simulink model "mcb_pmsm_param_est_host_f28379d"  (R2024b)
settings: Solver=FixedStepDiscrete  StartTime=0.0  StopTime=inf  RelTol=1e-3  EnableMultiTasking=on
StopFcn:
  | motorParam.p = motor.p;
  | motorParam.nomCurrent = motor.I_rated;
  | motorParam.PositionOffset = motor.PositionOffset;
  | motorParam.QEPSlits = motor.QEPSlits;
  | mcb_param_est_StopFunc(bdroot);
values from neighbouring files (symbols this model uses):
  Ts = T_pwm    (= 5e-05)    [mcb_pmsm_param_est_f28379d_data.m]
undefined symbols (not defined in the file or in its folder): motor
libraries: simulink x4, instrumentseriallib x3, mcbpmsmparamestlib x1
settings Model: Creator=The MathWorks, Inc.  LastModifiedBy=The MathWorks, Inc.
settings SolverCC: AlgebraicLoopSolver=TrustRegion
settings DataIOCC: LimitDataPoints=on  SaveFormat=Array  ReturnWorkspaceOutputs=off
settings OptimizationCC: ReuseModelBlockBuffer=off  LifeSpan=1  EfficientTunableParamExpr=on
settings DebuggingCC: UnderspecifiedInitializationDetection=Classic  MergeDetectMultiDrivingBlocksExec=none  SolverPrmCheckMsg=warning  ParameterPrecisionLossMsg=none  UnconnectedInputMsg=warning  UnconnectedOutputMsg=warning  UnconnectedLineMsg=warning  AllowSymbolicDim=off  PregeneratedLibrarySubsystemCodeDiagnostic=none  SubsystemReferenceDiagnosticForUnitTest=warning  SFUnexpectedBacktrackingDiag=warning  SFNoUnconditionalDefaultTransitionDiag=warning  SFExecutionAtInitializationDiag=none  ArithmeticOperatorsInVariantConditions=warning
settings HardwareCC: ProdBitPerPointer=32  ProdLargestAtomicFloat=None  ProdIntDivRoundTo=Undefined  ProdEndianess=Unspecified  ProdWordSize=32  ProdHWDeviceType=32-bit Generic
settings ModelReferenceCC: EnableRefExpFcnMdlSchedulingChecks=on  PropagateSignalLabelsOutOfModel=off
settings SFSimCC: SimUseLocalCustomCode=off  MATLABDynamicMemAlloc=off
settings RTWCC: Description=Real-Time Workshop Embedded Coder  SystemTargetFile=ert.tlc  TemplateMakefile=ert_default_tmf  GenerateReport=on  RTWUseLocalCustomCode=off  IncludeHyperlinkInReport=on  LaunchReport=on  GenerateTraceInfo=on  GenerateTraceReport=on  GenerateTraceReportSl=on  GenerateTraceReportSf=on  GenerateTraceReportEml=on  GPUComputeCapability=3.5  DLArmComputeVersion=19.05
settings CodeAppCC: IgnoreCustomStorageClasses=off  StateflowObjectComments=on  InternalIdentifier=Classic
settings ERTTargetCC: MultiwordLength=2048  GenerateSampleERTMain=on  InlinedParameterPlacement=Hierarchical  ERTCustomFileTemplate=example_file_process.tlc  ConvertIfToSwitch=off  SuppressUnreachableDefaultCases=off  DynamicArrayContainerType=coder::array
settings ConfigComp: CovMetricSettings=dw  CovSaveCumulativeToWorkspaceVar=on  CovSaveSingleToWorkspaceVar=on  CovExternalEMLEnable=off  CovSFcnEnable=off

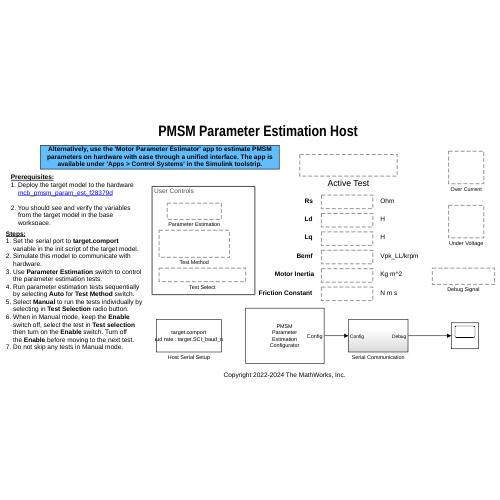
[thumbnail: Simulink's stored preview of the top-level diagram]
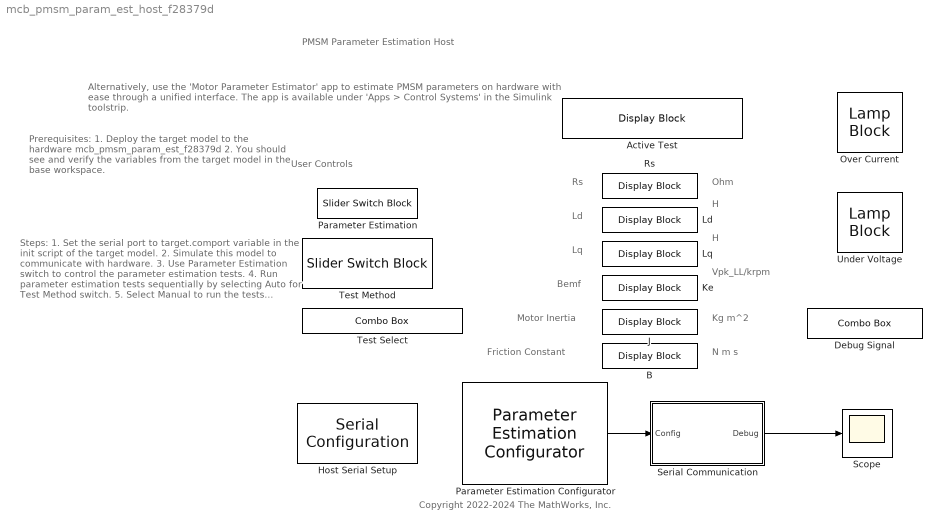
== system mcb_pmsm_param_est_host_f28379d ==
  note: Friction Constant
  note: User Controls
  note: PMSM Parameter Estimation Host
  note: Steps:
      | 1. Set the serial port to target.comport
      | variable in the init script of the target model.
      | 2. Simulate this model to communicate with
      | hardware.
      | 3. Use Parameter Estimation switch to control
      | the parameter estimation tests.
      | 4. Run parameter estimation tests sequentially
      | by selecting Auto for Test Method switch.
      | 5. Select Manual to run the tests individually by
      | selecting in Test Selection radio button.
      | 6. When in Manual mode, keep the Enable
      | switch off, select the test in Test selection
      | then turn on the Enable switch. Turn off
      | the Enable before moving to the next test.
      | 7. Do not skip any tests in Manual mode.
  note: H
  note: N m s
  note: Bemf
  note: Vpk_LL/krpm
  note: H
  note: Ohm
  note: Lq
  note: Rs
  note: Motor Inertia
  note: Copyright 2022-2024 The MathWorks, Inc.
  note: Ld
  note: Prerequisites:
      | 1. Deploy the target model to the hardware
      | mcb_pmsm_param_est_f28379d
      |
      | 2. You should see and verify the variables
      | from the target model in the base
      | workspace.
  note: Kg m^2
  note: Alternatively, use the 'Motor Parameter Estimator' app to estimate PMSM parameters on hardware with ease through a unified interface. The app is available under 'Apps > Control Systems' in the Simulink toolstrip.
  Active Test : DisplayBlock  LabelPosition=Hide  Transparency=1
  B : DisplayBlock  LabelPosition=Hide  Transparency=1
  Debug Signal : ComboBox  LabelPosition=Hide  SelectedLabel=Ia
      settings: Values={{'Ia', 'Ib', 'Vdc', 'Speed', 'Theta', 'Id', 'Iq', 'Vd', 'Vq', 'InjFreq', 'PhaseDiff', 'CoastDown Time'}, [1 2 3 4 5 6 7 8 9 10 11 12]}
  Host Serial Setup : instrumentseriallib/Serial Configuration  Priority=-99  PortSel=target.comport  Port=target.comport  ComPort=target.comport  BaudRate=target.SCI_baud_rate  DataBits=8  Parity=none  StopBits=1  ByteOrder=little-endian  FlowControl=none  Timeout=2  SimulateUsing=Interpreted execution  BlockInModel=on  aMode=5
      settings: LibrarySourceBlock=mcblib/Protection and Diagnostics/Host Serial Setup
  J : DisplayBlock  LabelPosition=Hide  Transparency=1
  Ke : DisplayBlock  LabelPosition=Hide  Transparency=1
  Ld : DisplayBlock  LabelPosition=Hide  Transparency=1
  Lq : DisplayBlock  LabelPosition=Hide  Transparency=1
  Over Current : LampBlock  LabelPosition=Hide
  Parameter Estimation : SliderSwitchBlock  LabelPosition=Hide
      settings: Values={{'Stop', 'Start'}, [0 1]}
  Parameter Estimation Configurator : mcbpmsmparamestlib/Parameter Estimation Configurator  P=motor.p  NRated=motor.N_rated  IRated=motor.I_rated  ImaxInverter=inverter.ISenseMax  RBoard=inverter.R_board  ISenseGain=0.0105  VSenseGain=0.0098  FreqMax=1000  FreqMin=400  FreqStepSweep=100  FreqStepEst=10  FreqNum=10  CurrMeasDelay=2 * 50e-6  KeTime=5  KeSpeed=0.9 * motor.N_rated  IqRefFOC=0.2  KpKiInputEnable=off  Kp=1  Ki=10  JSpeedLow=0.2 * motor.N_rated  DataType=single  Ts=Ts
      settings: LibrarySourceBlock=mcblib/Parameter Estimation/PMSM Parameter Estimation/Parameter Estimation Configurator
  Rs : DisplayBlock  LabelPosition=Hide  Transparency=1
  Scope : Scope
  Serial Communication : Subsystem
  Test Method : SliderSwitchBlock  LabelPosition=Hide
      settings: Values={{'Manual', 'Auto'}, [0 1]}
  Test Select : ComboBox  LabelPosition=Hide  SelectedLabel=No Test
      settings: Values={{'No Test', 'Rs', 'Ld', 'Lq', 'Ke, J, B'}, [0 1 2 3 4]}
  Under Voltage : LampBlock  LabelPosition=Hide
  wires:
  Serial Communication/1(Debug) -> Scope/1
  Parameter Estimation Configurator/1 -> Serial Communication/1(Config)

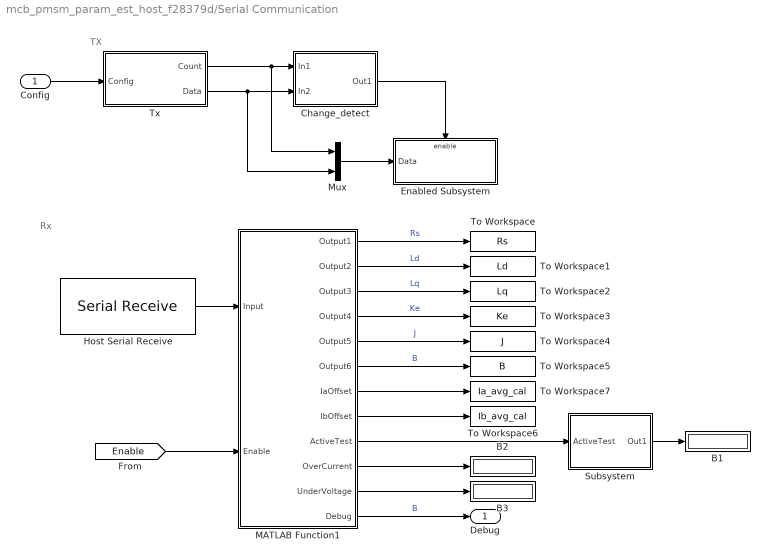
== system mcb_pmsm_param_est_host_f28379d/Serial Communication ==
  note: Rx
  note: TX
  Config : Inport
  B1 : Display
  B2 : Display
  B3 : Display
  Change_detect : Subsystem
  Enabled Subsystem : Subsystem  TreatAsAtomicUnit=on
  Host Serial Receive : instrumentseriallib/Serial Receive  PortSel=target.comport  Port=target.comport  ComPort=target.comport  DataType=single  SaveDataType=uint8  ToggleHeader=on  Header='SSSS'  ToggleDataSize=on  DataSize=[600 2]  ToggleTerminator=on  Terminator=Custom terminator  CustomTerminator='EEEE'  InputFormat=Row major  EnableBlockingMode=on  ActionDataUnavailable=Output custom value  ActionWhenDataUnavailable=Output custom value  CustomValue=4  SampleTime=600*Ts  SimulateUsing=Interpreted execution  BlockInModel=on  aMode=5
      settings: LibrarySourceBlock=mcblib/Protection and Diagnostics/Host Serial Receive
  MATLAB Function1 : MATLAB Function  TreatAsAtomicUnit=on
  Mux : Mux  Inputs=2
  Subsystem : Subsystem
  To Workspace : ToWorkspace  VariableName=Rs  SampleTime=-1
      settings: MaxDataPoints=1  Save2DSignal=2-D array (concatenate along first dimension)
  To Workspace1 : ToWorkspace  VariableName=Ld  SampleTime=-1
      settings: MaxDataPoints=1  Save2DSignal=2-D array (concatenate along first dimension)
  To Workspace2 : ToWorkspace  VariableName=Lq  SampleTime=-1
      settings: MaxDataPoints=1  Save2DSignal=2-D array (concatenate along first dimension)
  To Workspace3 : ToWorkspace  VariableName=Ke  SampleTime=-1
      settings: MaxDataPoints=1  Save2DSignal=2-D array (concatenate along first dimension)
  To Workspace4 : ToWorkspace  VariableName=J  SampleTime=-1
      settings: MaxDataPoints=1  Save2DSignal=2-D array (concatenate along first dimension)
  To Workspace5 : ToWorkspace  VariableName=B  SampleTime=-1
      settings: MaxDataPoints=1  Save2DSignal=2-D array (concatenate along first dimension)
  To Workspace6 : ToWorkspace  VariableName=Ib_avg_cal  SampleTime=-1
      settings: MaxDataPoints=1  Save2DSignal=2-D array (concatenate along first dimension)
  To Workspace7 : ToWorkspace  VariableName=Ia_avg_cal  SampleTime=-1
      settings: MaxDataPoints=1  Save2DSignal=2-D array (concatenate along first dimension)
  Tx : Subsystem
  Debug : Outport
  wires:
  Host Serial Receive/1 -> MATLAB Function1/1(Input)
  Change_detect/1(Out1) -> Enabled Subsystem/Enable
  Tx/1(Count) -> Mux/1, Change_detect/1(In1)
  Tx/2(Data) -> Mux/2, Change_detect/2(In2)
  Mux/1 -> Enabled Subsystem/1(Data)
  MATLAB Function1/1(Output1) -> To Workspace/1  "Rs"
  MATLAB Function1/2(Output2) -> To Workspace1/1  "Ld"
  MATLAB Function1/3(Output3) -> To Workspace2/1  "Lq"
  MATLAB Function1/4(Output4) -> To Workspace3/1  "Ke"
  MATLAB Function1/5(Output5) -> To Workspace4/1  "J"
  MATLAB Function1/6(Output6) -> To Workspace5/1  "B"
  Config/1 -> Tx/1(Config)
  MATLAB Function1/12(Debug) -> Debug/1  "B"
  MATLAB Function1/10(OverCurrent) -> B2/1
  MATLAB Function1/11(UnderVoltage) -> B3/1
  MATLAB Function1/9(ActiveTest) -> Subsystem/1(ActiveTest)
  Subsystem/1(Out1) -> B1/1
  MATLAB Function1/7(IaOffset) -> To Workspace7/1
  MATLAB Function1/8(IbOffset) -> To Workspace6/1
  [Enable] -> MATLAB Function1/2(Enable)

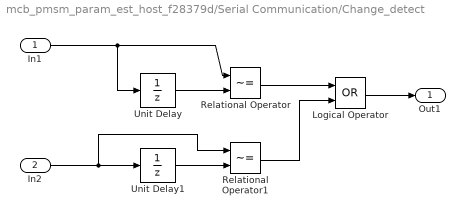
== system mcb_pmsm_param_est_host_f28379d/Serial Communication/Change_detect ==
  In1 : Inport
  In2 : Inport  Port=2
  Logical Operator : Logic  Operator=OR  AllPortsSameDT=off  OutDataTypeStr=boolean
  Relational Operator : RelationalOperator  Operator=~=  OutDataTypeStr=boolean  InputSameDT=off
  Relational Operator1 : RelationalOperator  Operator=~=  OutDataTypeStr=boolean  InputSameDT=off
  Unit Delay : UnitDelay  InitialCondition=0.5  SampleTime=-1  HasFrameUpgradeWarning=on
  Unit Delay1 : UnitDelay  SampleTime=-1  HasFrameUpgradeWarning=on
  Out1 : Outport  VectorParamsAs1DForOutWhenUnconnected=off
  wires:
  In2/1 -> Relational Operator1/1, Unit Delay1/1
  Relational Operator1/1 -> Logical Operator/2
  Unit Delay1/1 -> Relational Operator1/2
  Unit Delay/1 -> Relational Operator/2
  In1/1 -> Unit Delay/1, Relational Operator/1
  Relational Operator/1 -> Logical Operator/1
  Logical Operator/1 -> Out1/1

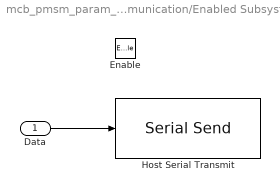
== system mcb_pmsm_param_est_host_f28379d/Serial Communication/Enabled Subsystem ==
  Data : Inport
  Enable : EnablePort
  Host Serial Transmit : instrumentseriallib/Serial Send  PortSel=target.comport  Port=target.comport  ComPort=target.comport  Header=[]  Terminator=<none>  CustomTerminator=[]  EnableBlockingMode=off  SimulateUsing=Interpreted execution  BlockInModel=on  aMode=5
      settings: LibrarySourceBlock=mcblib/Protection and Diagnostics/Host Serial Transmit
  wires:
  Data/1 -> Host Serial Transmit/1

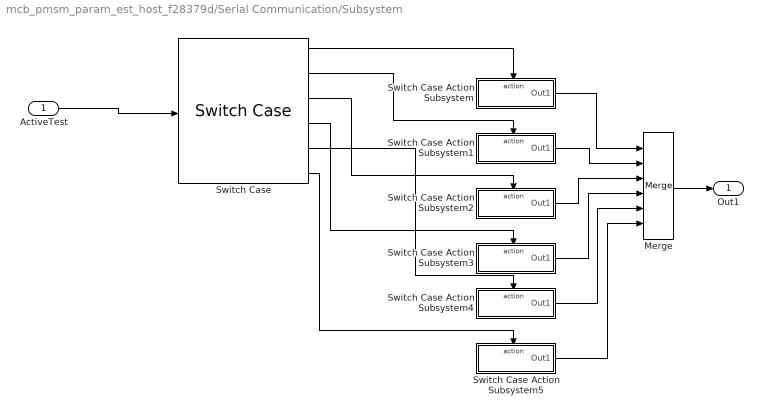
== system mcb_pmsm_param_est_host_f28379d/Serial Communication/Subsystem ==
  ActiveTest : Inport
  Merge : Merge  Inputs=6
  Switch Case : SwitchCase  CaseConditions={0,1,2,3,4}
  Switch Case Action Subsystem : Subsystem  TreatAsAtomicUnit=on
  Switch Case Action Subsystem1 : Subsystem  TreatAsAtomicUnit=on
  Switch Case Action Subsystem2 : Subsystem  TreatAsAtomicUnit=on
  Switch Case Action Subsystem3 : Subsystem  TreatAsAtomicUnit=on
  Switch Case Action Subsystem4 : Subsystem  TreatAsAtomicUnit=on
  Switch Case Action Subsystem5 : Subsystem  TreatAsAtomicUnit=on
  Out1 : Outport
  wires:
  Merge/1 -> Out1/1
  ActiveTest/1 -> Switch Case/1
  Switch Case/1 -> Switch Case Action Subsystem/Action
  Switch Case/2 -> Switch Case Action Subsystem1/Action
  Switch Case/3 -> Switch Case Action Subsystem2/Action
  Switch Case/4 -> Switch Case Action Subsystem3/Action
  Switch Case/5 -> Switch Case Action Subsystem4/Action
  Switch Case/6 -> Switch Case Action Subsystem5/Action
  Switch Case Action Subsystem1/1(Out1) -> Merge/2
  Switch Case Action Subsystem2/1(Out1) -> Merge/3
  Switch Case Action Subsystem/1(Out1) -> Merge/1
  Switch Case Action Subsystem3/1(Out1) -> Merge/4
  Switch Case Action Subsystem4/1(Out1) -> Merge/5
  Switch Case Action Subsystem5/1(Out1) -> Merge/6

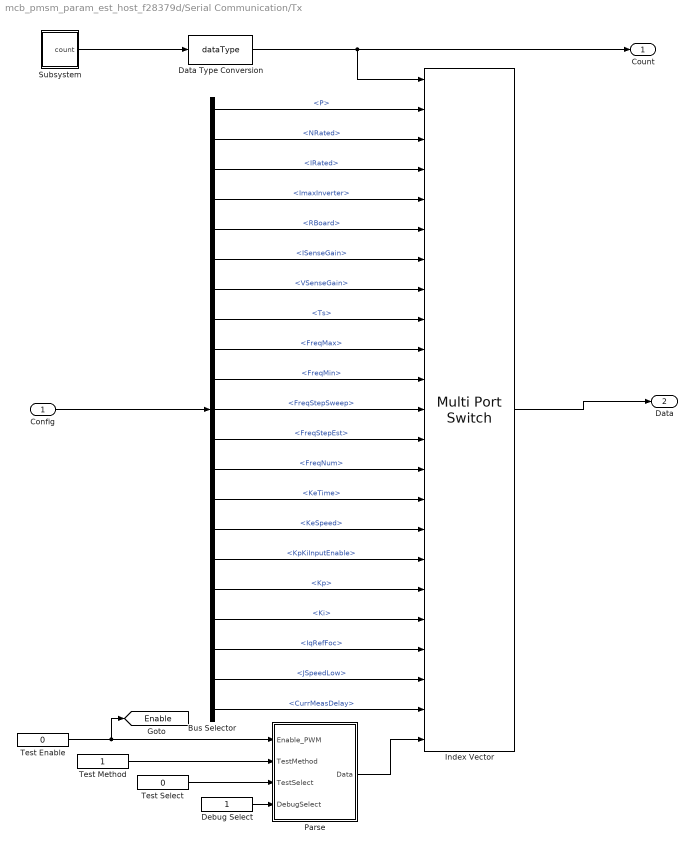
== system mcb_pmsm_param_est_host_f28379d/Serial Communication/Tx ==
  Config : Inport
  Bus Selector : BusSelector  OutputSignals=P,NRated,IRated,ImaxInverter,RBoard,ISenseGain,VSenseGain,Ts,FreqMax,FreqMin,FreqStepSweep,FreqStepEst,FreqNum,KeTime,KeSpeed,KpKiInputEnable,Kp,Ki,IqRefFoc,JSpeedLow,CurrMeasDelay
  Data Type Conversion : DataTypeConversion  OutDataTypeStr=dataType  RndMeth=Simplest  SaturateOnIntegerOverflow=off
  Debug Select : Constant  OutDataTypeStr=uint16  SampleTime=600 * Ts
  Index Vector : MultiPortSwitch  Inputs=22  OutDataTypeStr=dataType  RndMeth=Simplest  SaturateOnIntegerOverflow=off  InputSameDT=off
  Parse : Subsystem
  Subsystem : Subsystem  mask(Counter){upperLimit=22, sampleTime=600 * Ts}
      mask prompts: upperLimit "Upper Limit"; sampleTime "Sample Time"
      mask help: Conter starts from 1 and reaches Upper Limit using given sample time in steps of 1.
  Test Enable : Constant  Value=0  VectorParams1D=off  OutDataTypeStr=uint16  SampleTime=600 * Ts
  Test Method : Constant  VectorParams1D=off  OutDataTypeStr=uint16  SampleTime=600 * Ts
  Test Select : Constant  Value=0  OutDataTypeStr=uint16  SampleTime=600 * Ts
  Count : Outport
  Data : Outport  Port=2
  tag scope: Enable=global
  wires:
  Bus Selector/20 -> Index Vector/21  "<JSpeedLow>"
  Bus Selector/19 -> Index Vector/20  "<IqRefFoc>"
  Bus Selector/18 -> Index Vector/19  "<Ki>"
  Bus Selector/17 -> Index Vector/18  "<Kp>"
  Bus Selector/16 -> Index Vector/17  "<KpKiInputEnable>"
  Bus Selector/15 -> Index Vector/16  "<KeSpeed>"
  Bus Selector/14 -> Index Vector/15  "<KeTime>"
  Bus Selector/13 -> Index Vector/14  "<FreqNum>"
  Bus Selector/12 -> Index Vector/13  "<FreqStepEst>"
  Bus Selector/11 -> Index Vector/12  "<FreqStepSweep>"
  Bus Selector/10 -> Index Vector/11  "<FreqMin>"
  Bus Selector/9 -> Index Vector/10  "<FreqMax>"
  Bus Selector/8 -> Index Vector/9  "<Ts>"
  Bus Selector/7 -> Index Vector/8  "<VSenseGain>"
  Bus Selector/6 -> Index Vector/7  "<ISenseGain>"
  Bus Selector/5 -> Index Vector/6  "<RBoard>"
  Bus Selector/4 -> Index Vector/5  "<ImaxInverter>"
  Bus Selector/3 -> Index Vector/4  "<IRated>"
  Bus Selector/2 -> Index Vector/3  "<NRated>"
  Bus Selector/1 -> Index Vector/2  "<P>"
  Test Enable/1 -> Parse/1(Enable_PWM), [Enable]
  Debug Select/1 -> Parse/4(DebugSelect)
  Data Type Conversion/1 -> Count/1, Index Vector/1
  Index Vector/1 -> Data/1
  Subsystem/1(count) -> Data Type Conversion/1
  Test Method/1 -> Parse/2(TestMethod)
  Test Select/1 -> Parse/3(TestSelect)
  Config/1 -> Bus Selector/1
  Bus Selector/21 -> Index Vector/22  "<CurrMeasDelay>"
  Parse/1(Data) -> Index Vector/23

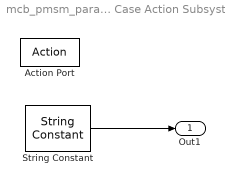
== system mcb_pmsm_param_est_host_f28379d/Serial Communication/Subsystem/Switch Case Action Subsystem ==
  Action Port : ActionPort  ActionPortLabel=case [ 0 ]:
  String Constant : StringConstant  String="\"Inactive\""
  Out1 : Outport
  wires:
  String Constant/1 -> Out1/1

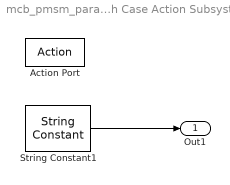
== system mcb_pmsm_param_est_host_f28379d/Serial Communication/Subsystem/Switch Case Action Subsystem1 ==
  Action Port : ActionPort  ActionPortLabel=case [ 1 ]:
  String Constant1 : StringConstant  String="\"Rs Test\""
  Out1 : Outport
  wires:
  String Constant1/1 -> Out1/1

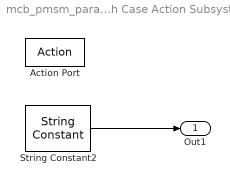
== system mcb_pmsm_param_est_host_f28379d/Serial Communication/Subsystem/Switch Case Action Subsystem2 ==
  Action Port : ActionPort  ActionPortLabel=case [ 2 ]:
  String Constant2 : StringConstant  String="\"Ld Test\""
  Out1 : Outport
  wires:
  String Constant2/1 -> Out1/1

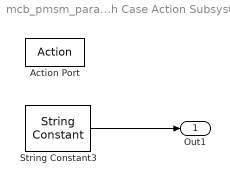
== system mcb_pmsm_param_est_host_f28379d/Serial Communication/Subsystem/Switch Case Action Subsystem3 ==
  Action Port : ActionPort  ActionPortLabel=case [ 3 ]:
  String Constant3 : StringConstant  String="\"Lq Test\""
  Out1 : Outport
  wires:
  String Constant3/1 -> Out1/1

== system mcb_pmsm_param_est_host_f28379d/Serial Communication/Subsystem/Switch Case Action Subsystem4 ==
  Action Port : ActionPort  ActionPortLabel=case [ 4 ]:
  String Constant4 : StringConstant  String="\"Ke, J, B Test\""
  Out1 : Outport
  wires:
  String Constant4/1 -> Out1/1

== system mcb_pmsm_param_est_host_f28379d/Serial Communication/Subsystem/Switch Case Action Subsystem5 ==
  Action Port : ActionPort  ActionPortLabel=default:
  String Constant : StringConstant  String="\"Inactive\""
  Out1 : Outport
  wires:
  String Constant/1 -> Out1/1

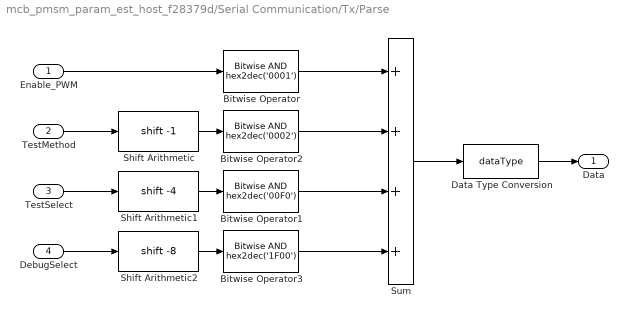
== system mcb_pmsm_param_est_host_f28379d/Serial Communication/Tx/Parse ==
  Enable_PWM : Inport
  TestMethod : Inport  Port=2
  TestSelect : Inport  Port=3
  DebugSelect : Inport  Port=4
  Bitwise Operator : simulink/Logic and Bit Operations/Bitwise Operator  logicop=AND  UseBitMask=on  BitMask=hex2dec('0001')  BitMaskRealWorld=Stored Integer
  Bitwise Operator1 : simulink/Logic and Bit Operations/Bitwise Operator  logicop=AND  UseBitMask=on  BitMask=hex2dec('00F0')  BitMaskRealWorld=Stored Integer
  Bitwise Operator2 : simulink/Logic and Bit Operations/Bitwise Operator  logicop=AND  UseBitMask=on  BitMask=hex2dec('0002')  BitMaskRealWorld=Stored Integer
  Bitwise Operator3 : simulink/Logic and Bit Operations/Bitwise Operator  logicop=AND  UseBitMask=on  BitMask=hex2dec('1F00')  BitMaskRealWorld=Stored Integer
  Data Type Conversion : DataTypeConversion  OutDataTypeStr=dataType  RndMeth=Simplest  SaturateOnIntegerOverflow=off
  Shift Arithmetic : ArithShift  BitShiftNumber=-1
  Shift Arithmetic1 : ArithShift  BitShiftNumber=-4
  Shift Arithmetic2 : ArithShift  BitShiftNumber=-8
  Sum : Sum  Inputs=++++
  Data : Outport
  wires:
  Bitwise Operator3/1 -> Sum/4
  Shift Arithmetic2/1 -> Bitwise Operator3/1
  DebugSelect/1 -> Shift Arithmetic2/1
  Data Type Conversion/1 -> Data/1
  Enable_PWM/1 -> Bitwise Operator/1
  Bitwise Operator2/1 -> Sum/2
  TestMethod/1 -> Shift Arithmetic/1
  Bitwise Operator1/1 -> Sum/3
  Shift Arithmetic/1 -> Bitwise Operator2/1
  Shift Arithmetic1/1 -> Bitwise Operator1/1
  Sum/1 -> Data Type Conversion/1
  TestSelect/1 -> Shift Arithmetic1/1
  Bitwise Operator/1 -> Sum/1

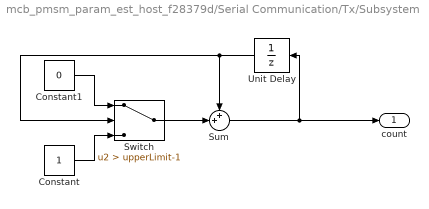
== system mcb_pmsm_param_est_host_f28379d/Serial Communication/Tx/Subsystem ==
  Constant : Constant  OutDataTypeStr=uint8  SampleTime=sampleTime
  Constant1 : Constant  Value=0  OutDataTypeStr=uint8  SampleTime=sampleTime
  Sum : Sum  Inputs=++|  OutDataTypeStr=uint8  AccumDataTypeStr=uint8  RndMeth=Simplest
  Switch : Switch  Criteria=u2 > Threshold  Threshold=upperLimit-1  OutDataTypeStr=uint8  RndMeth=Simplest  SaturateOnIntegerOverflow=off  InputSameDT=off
  Unit Delay : UnitDelay  SampleTime=-1  HasFrameUpgradeWarning=on
  count : Outport
  wires:
  Constant/1 -> Switch/3
  Switch/1 -> Sum/2
  Unit Delay/1 -> Sum/1, Switch/2
  Sum/1 -> Unit Delay/1, count/1
  Constant1/1 -> Switch/1

== matlab function mcb_pmsm_param_est_host_f28379d/Serial Communication/MATLAB Function1 ==
  data: Output1 output; Output2 output; Output3 output; Output4 output; Output5 output; Output6 output; IaOffset output; IbOffset output; ActiveTest output; OverCurrent output; UnderVoltage output; Debug output; Input input; Enable input
function [ Output1, Output2, Output3, Output4, Output5, Output6, IaOffset, IbOffset, ActiveTest,  OverCurrent, UnderVoltage, Debug] = unBuf(Input, Enable)

coder.extrinsic('message', 'msgbox', 'set_param', 'error');

Output1 = Input(1, 1);
Output2 = Input(2, 1);
Output3 = Input(3, 1);
Output4 = Input(4, 1);
Output5 = Input(5, 1);
Output6 = Input(6, 1);
IaOffset= Input(7, 1);
IbOffset= Input(8, 1);
ActiveTest = Input(9, 1);
OverCurrent = Input(10, 1);
UnderVoltage = Input(11, 1);
if (OverCurrent > 0 || UnderVoltage > 0) && Enable > 0
    set_param(bdroot, 'SimulationCommand','stop')
end
Debug = Input(:,2);

end
